simulink model "InverznaFunkcija"  (R2016b)
settings: Solver=VariableStepAuto  StartTime=0.0  StopTime=50  RelTol=1e-3
libraries: simulink x1
settings Model: Creator=Luka  LastModifiedBy=Luka

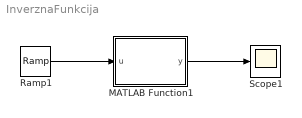
== system InverznaFunkcija ==
  MATLAB Function1 : MATLAB Function  TreatAsAtomicUnit=on
  Ramp1 : simulink/Sources/Ramp  slope=1  start=0  X0=0
  Scope1 : Scope
  wires:
  MATLAB Function1/1(y) -> Scope1/1
  Ramp1/1 -> MATLAB Function1/1(u)

== matlab function InverznaFunkcija/MATLAB Function1 ==
  data: u input; y output
function y = fcn(u)

y = -200*log(1 - u/50);
